simulink model "Cruise_Control"  (R2020a)
settings: Solver=ode45  StartTime=0.0  StopTime=120  RelTol=1e-3
values from neighbouring files (symbols this model uses):
  b = 50.0    [DD_Cruise_Control.sldd]
  m = 1000.0    [DD_Cruise_Control.sldd]
settings Model: DataDictionary=DD_Cruise_Control.sldd  Creator=Noel Varghese  LastModifiedBy=Noel Varghese
settings DataIOCC: SaveOutput=off  SaveTime=off

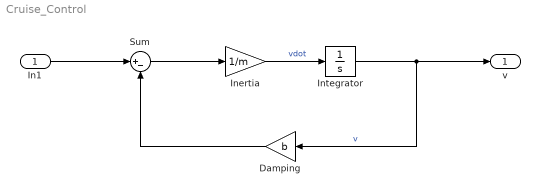
== system Cruise_Control ==
  In1 : Inport  OutDataTypeStr=double  PortDimensions=1  SampleTime=0
  Damping : Gain  Gain=b
  Inertia : Gain  Gain=1/m
  Integrator : Integrator
  Sum : Sum  Inputs=|+-
  v : Outport  OutDataTypeStr=double  PortDimensions=1  SampleTime=0
  wires:
  Inertia/1 -> Integrator/1  "vdot"
  Integrator/1 -> Damping/1, v/1  "v"
  In1/1 -> Sum/1
  Sum/1 -> Inertia/1
  Damping/1 -> Sum/2
